simulink model "MathematicalModel"  (R2024a)
settings: Solver=VariableStepAuto  StartTime=0.0  StopTime=10.0  RelTol=1e-3
values from neighbouring files (symbols this model uses):
  beta = 3.5    [values.m]
  g = 9.81    [values.m]
  h = H * 0.567    (= 0.9072)    [values.m]
  H = 1.60    (= 1.6)    [values.m]
  Is = m * (K*H).^2    [values.m]
  K = 0.448    [values.m]
  Tmus = 0.1    [values.m]
settings Model: Creator=franc  LastModifiedBy=franc

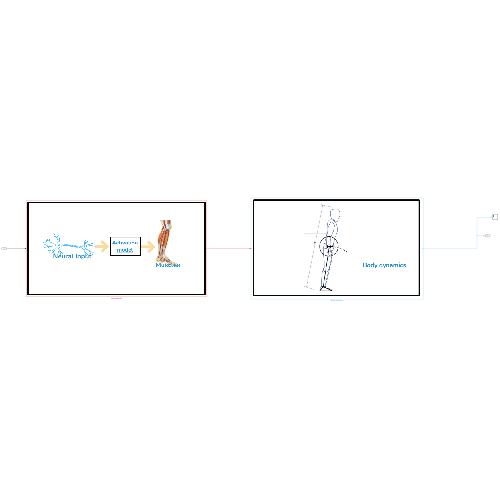
[thumbnail: Simulink's stored preview of the top-level diagram]
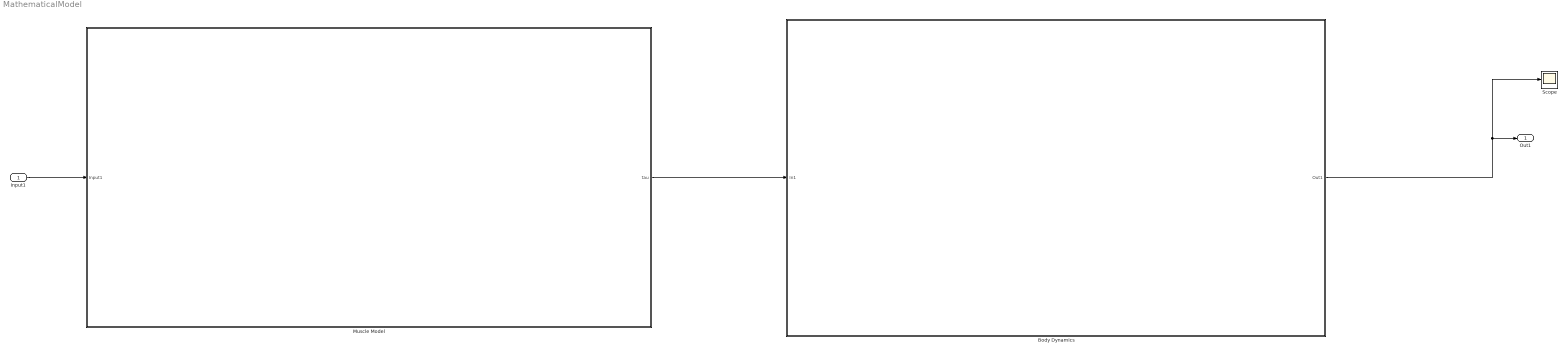
== system MathematicalModel ==
  Input1 : Inport
  Body Dynamics : Subsystem
      mask Display: image('body2.png');
  Muscle Model : Subsystem
      mask Display: image('muscleModel.png');
  Scope : Scope
  Out1 : Outport
  wires:
  Muscle Model/1(tau) -> Body Dynamics/1(In1)
  Body Dynamics/1(Out1) -> Scope/1, Out1/1
  Input1/1 -> Muscle Model/1(Input1)

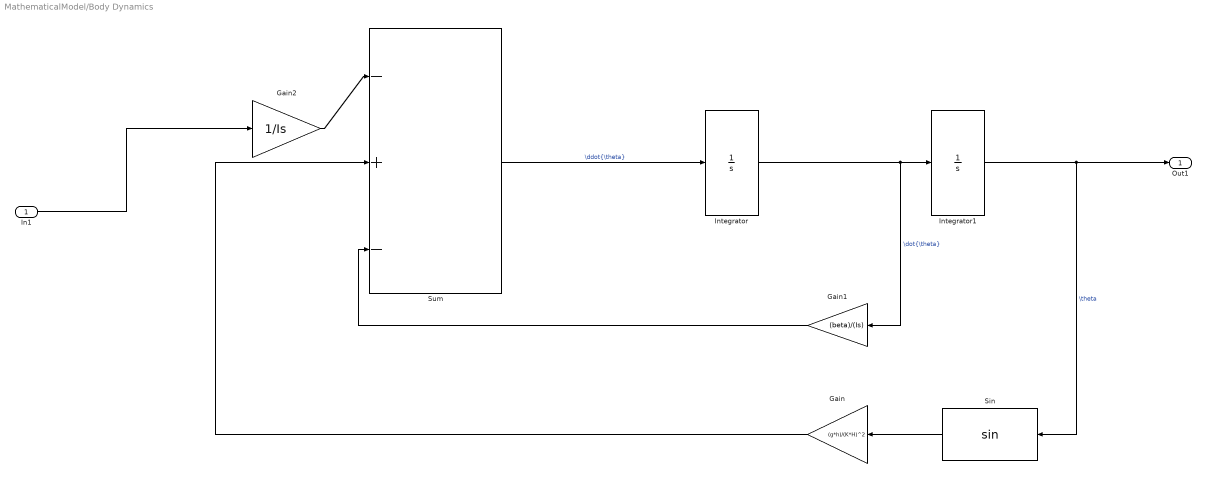
== system MathematicalModel/Body Dynamics ==
  In1 : Inport
  Gain : Gain  Gain=(g*h)/(K*H)^2
  Gain1 : Gain  Gain=(beta)/(Is)
  Gain2 : Gain  Gain=1/Is
  Integrator : Integrator
  Integrator1 : Integrator
  Sin : Trigonometry
  Sum : Sum  Inputs=|-+-
  Out1 : Outport
  wires:
  Sum/1 -> Integrator/1  "\\ddot{\\theta}"
  Integrator1/1 -> Out1/1, Sin/1  "\\theta"
  Gain1/1 -> Sum/3
  Integrator/1 -> Gain1/1, Integrator1/1  "\\dot{\\theta}"
  Sin/1 -> Gain/1
  Gain2/1 -> Sum/1
  Gain/1 -> Sum/2
  In1/1 -> Gain2/1

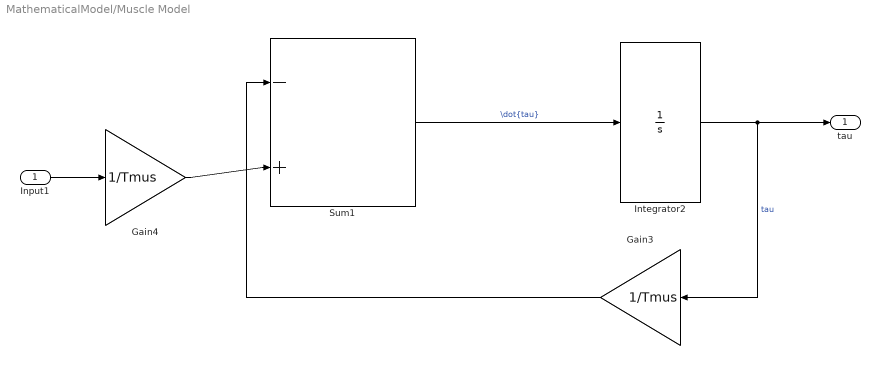
== system MathematicalModel/Muscle Model ==
  Input1 : Inport
  Gain3 : Gain  Gain=1/Tmus
  Gain4 : Gain  Gain=1/Tmus
  Integrator2 : Integrator
  Sum1 : Sum  Inputs=|-+
  tau : Outport
  wires:
  Gain3/1 -> Sum1/1
  Integrator2/1 -> tau/1, Gain3/1  "tau"
  Sum1/1 -> Integrator2/1  "\\dot{tau}"
  Input1/1 -> Gain4/1
  Gain4/1 -> Sum1/2
